simulink model "sm_water_powered_lift"  (R2026a)
settings: Solver=ode15s  StopTime=50  MaxStep=1e-2  AbsTol=1e-4  EnableMultiTasking=on
undefined symbols (not defined in the file or in its folder): wrat, X, Y, Z
libraries: sm_lib x47, nesl_utility x13, fl_lib x10, Multibody_Parts_Lib x2, simulink x1
(part 1 of 2)
CloseFcn:
  | try,close(h1_sm_water_powered_lift),end
  | clear h1_sm_water_powered_lift
  | 
  | clear simlog_sm_water_powered_lift
  | clear logsout_sm_water_powered_lift
Description:
  | Water Powered Lift
  | 
  | Copyright 2017-2026 The MathWorks, Inc.
settings Model: Tag=PublishSubsystem  Creator=smiller  LastModifiedBy=smiller
settings DataIOCC: MaxDataPoints=15000  SignalLoggingName=logsout_sm_water_powered_lift
settings DebuggingCC: PregeneratedLibrarySubsystemCodeDiagnostic=none
settings SimscapeCC: SimscapeNormalizeSystem=off  SimscapeNominalValues="[{\"value\":\"1\",\"unit\":\"A\"},{\"value\":\"1\",\"unit\":\"bar\"},{\"value\":\"1\",\"unit\":\"cm^2\"},{\"value\":\"1\",\"unit\":\"cm^3/s\"},{\"value\":\"1\",\"unit\":\"kJ/kg\"},{\"value\":\"1\",\"unit\":\"kW\"},{\"value\":\"1\",\"unit\":\"l\"},{\"value\":\"1\",\"unit\":\"N\"},{\"value\":\"1\",\"unit\":\"N*m\"},{\"value\":\"1\",\"unit\":\"V\"}]"  SimscapeLogSimulationStatistics=on  SimscapeLogName=simlog_sm_water_powered_lift  SimscapeLogDataHistory=15000.0
settings ConfigurationSet: Description=SimMechanics 2G
settings ExplorerConfigSet: InternalSimMechanicsExplorerSettings="<ExplorerConfiguration><canonicalview>default</canonicalview><AnimationSetting><BasePlaybackSpeed>1.0</BasePlaybackSpeed><PlaybackSpeedFactor>2.0</PlaybackSpeedFactor></AnimationSetting><TilePanel><TileInfo><Tiles Columns=\"2\" Count=\"4\" Rows=\"2\"><Column Left=\"2\" Weight=\"0.4992\"/><Column Left=\"314\" Weight=\"0.5008\"/><Column Left=\"627\"/><Row Top=\"2\" Weight=\"0.4993\"/><Row Top=\"345\" Weight=\"0.5007\"/><Row Top=\"689\"/><Tile Height=\"1\" Width=\"1\" X=\"0\" Y=\"0\"/><Tile Height=\"1\" Width=\"1\" X=\"0\" Y=\"1\"/><Tile Height=\"1\" Width=\"1\" X=\"1\" Y=\"0\"/><Tile Height=\"1\" Width=\"1\" X=\"1\" Y=\"1\"/></Tiles></TileInfo><SceneInfo><SceneViewer><BGColor><R>1</R><G>1</G><B>1</B></BGColor><Camera><DoPerspective>off</DoPerspective><Position><X>-0.33865632822427127</X><Y>-0.74181965766312075</Y><Z>0.63517646256957694</Z></Position><Center><X>0.17435806215764543</X><Y>0.41659149528563333</Y><Z>0.46311042540191633</Z></Center><Up><X>0.044233510300130147</X><Y>0.12758646822646313</Y><Z>0.99084059751910947</Z></Up><ViewLimDist>1</ViewLimDist><YLim>0.73418943875669118</YLim><XLim>0.66604610761460303</XLim></Camera></SceneViewer><SceneViewer><BGColor><R>1</R><G>1</G><B>1</B></BGColor><Camera><DoPerspective>on</DoPerspective><Position><X>-0.36750000000000016</X><Y>0.94385156136048332</Y><Z>0.52251828153286128</Z></Position><Center><X>-0.12000000000000008</X><Y>0.94875767701724301</Y><Z>0.32382884414586155</Z></Center><Up><X>0</X><Y>0</Y><Z>1</Z></Up><ViewLimDist>1</ViewLimDist><YLim>0.46630765815499858</YLim><XLim>0.42176483707750617</XLim></Camera></SceneViewer><SceneViewer><BGColor><R>1</R><G>1</G><B>1</B></BGColor><Camera><DoPerspective>off</DoPerspective><Position><X>-0.8984869340885806</X><Y>0.0036381965185360507</Y><Z>0.11209190037180658</Z></Position><Center><X>0.20238156217890113</X><Y>0.0036381965185360507</Y><Z>0.11209190037180658</Z></Center><Up><X>0</X><Y>0</Y><Z>1</Z></Up><ViewLimDist>1</ViewLimDist><YLim>0.37360343949453689</YLim><XLim>0.34004624433035691</XLim></Camera></SceneViewer><SceneViewer><BGColor><R>1</R><G>1</G><B>1</B></BGColor><Camera><DoPerspective>on</DoPerspective><Position><X>0.10106831738082762</X><Y>-0.30413148543864094</Y><Z>0.35203766090491534</Z></Position><Center><X>0.3950004490262965</X><Y>-0.032632326314832705</Y><Z>0.15132570006540724</Z></Center><Up><X>0.30158145199882502</X><Y>0.33375611692514179</Y><Z>0.89311560406552715</Z></Up><ViewLimDist>1</ViewLimDist><YLim>0.46630765815499858</YLim><XLim>0.42315680023617785</XLim></Camera></SceneViewer></SceneInfo></TilePanel><MechEditorPanel><Cameras><Camera><Id>Camera1</Id><Value><Name>Bucket</Name><NativeCamera><PositionTrackingFeature>Arm.Bucket.Transform_Camera.F</PositionTrackingFeature><CenterTrackingFeature>Arm.Arm.Pin_Side_1.Frame1</CenterTrackingFeature><UpVectorTrackingFeature>World_Frame.W</UpVectorTrackingFeature><CenterTrackingOrigin>on</CenterTrackingOrigin><UpVectorTrackingDirection>+Z</UpVectorTrackingDirection></NativeCamera></Value></Camera><Camera><Id>Camera2</Id><Value><Name>Gear</Name><NativeCamera><PositionKeyframeSet><Keyframe><Time>+0.0000000000000000e+00</Time><Value><X>+1.0106831738082762e-01</X><Y>-3.0413148543864094e-01</Y><Z>+3.5203766090491534e-01</Z></Value></Keyframe></PositionKeyframeSet><CenterKeyframeSet><Keyframe><Time>+0.0000000000000000e+00</Time><Value><X>+3.9500044902629650e-01</X><Y>-3.2632326314832705e-02</Y><Z>+1.5132570006540724e-01</Z></Value></Keyframe></CenterKeyframeSet><UpVectorKeyframeSet><Keyframe><Time>+0.0000000000000000e+00</Time><Value><X>+3.0158145199882502e-01</X><Y>+3.3375611692514179e-01</Y><Z>+8.9311560406552715e-01</Z></Value></Keyframe></UpVectorKeyframeSet></NativeCamera></Value></Camera></Cameras><GfxPanelCameraMap><MapElement CameraMLId=\"Camera1\" GfxPanelIndex=\"1\"/><MapElement CameraMLId=\"Camera2\" GfxPanelIndex=\"3\"/></GfxPanelCameraMap><VideoCreator><PlaybackSpeedRatio>1.0</PlaybackSpeedRatio><FrameRate>30</FrameRate><VideoFormat>Motion JPEG AVI</VideoFormat><FrameSize>auto</FrameSize></VideoCreator></MechEditorPanel></ExplorerConfiguration>"

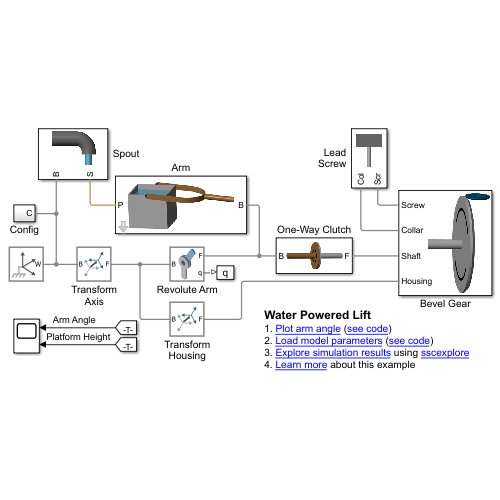
[thumbnail: Simulink's stored preview of the top-level diagram]
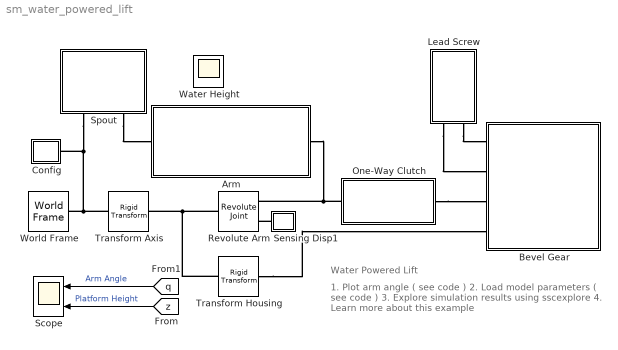
== system sm_water_powered_lift ==
  note: Water Powered Lift
  note: 1. Plot arm angle ( see code )
      | 2. Load model parameters ( see code )
      | 3. Explore simulation results using sscexplore
      | 4. Learn more about this example
  Arm : Subsystem  mask(Water Wheel Arm with Bucket){spoke_angle=30, spoke_length=wrat.spoke.length, spoke_radius=wrat.spoke.radius, spoke_angle_fill=-[40 55], bracket_rad=wrat.bracket.radius, bracket_height=wrat.bracket.height, bracket_thickness=wrat.bracket.thickness, bracket_sidelen=wrat.bracket.side.length, arc_xc=wrat.bracket.extr_data, whl_rho=wrat.wheel.rho, whl_clr=wrat.wheel.color, bucket_side=wrat.bucket.side, bucket_height=wrat.bucket.height, bucket_hole_side=wrat.bucket.hole.side, pin_viscfrict=wrat.bucket.pin_friction, bucket_rho=wrat.bucket.rho, bucket_wallthickness=wrat.bucket.wall_thickness, bucket_clr=wrat.bucket.color, bucket_opc=wrat.bucket.opacity*0.5, water_rho=wrat.water.rho, check_wlevel=off, water_clr_level=wrat.water.clr, water_opc_level=wrat.water.opc, water_thickness_level=wrat.water.surface_thickness, check_wellip=off, water_clr_ellip=wrat.water.clr, water_opc_ellip=wrat.water.opc}
      mask prompts: spoke_angle "Angle (deg)"; spoke_length "Length (m)"; spoke_radius "Radius (m)"; spoke_angle_fill "Angle Range for Fill [min max] (deg)"; bracket_rad "Radius (m)"; bracket_height "Height (m)"; bracket_thickness "Thickness (m)"; bracket_sidelen "Side Length (m)"; arc_xc "Arc Cross Section [xy] (m)"; whl_rho "Density (kg/m^3)"; whl_clr "Color [RGB]"; bucket_side "Side Length (m)"; bucket_height "Height (m)"; bucket_hole_side "Hole Side Length (m)"; pin_viscfrict "Friction at Pin (N*m/(deg/s))"; bucket_rho "Density (kg/m^3)"; bucket_wallthickness "Wall Thickness (m)"; bucket_clr "Color [RGB]"; bucket_opc "Opacity (0-1)"; water_rho "Density (kg/m^3)"; check_wlevel "Show Water Level"; water_clr_level "Color [RGB]"; water_opc_level "Opacity (0-1)"; water_thickness_level "Surface thickness (m)"; check_wellip "Show Water Inertia Ellipsoid"; water_clr_ellip "Color [RGB]"; water_opc_ellip "Opacity (0-1)"
      mask help: Models a single spoke of a water wheel with a bucket at the end. Multibody port B is the axis end of the arm. Inport Flow is the volumetric flow of water in kg^3/s.
      mask init:
      | bucket_wall_xc =[
      |     bucket_side/2  bucket_side/2;
      |     -bucket_side/2  bucket_side/2;
      |     -bucket_side/2  -bucket_side/2;
      |     bucket_side/2  -bucket_side/2;
      |     bucket_side/2  bucket_side/2;
      |     bucket_side/2-bucket_wallthickness  bucket_side/2-bucket_wallthickness;
      |     bucket_side/2-bucket_wallthickness  -(bucket_side/2-bucket_wallthickness);
      |     -(bucket_side/2-bucket_wallthickness)  -(bucket_side/2-bucket_wallthickness);
      |     -(bucket_side/2-bucket_wallthickness)  (bucket_side/2-bucket_wallthickness);
      |     (bucket_side/2-bucket_wallthickness)  (bucket_side/2-bucket_wallthickness)];
      | 
      | bucket_floor_xc = [
      |     bucket_side/2  bucket_side/2;
      |     -bucket_side/2  bucket_side/2;
      |     -bucket_side/2  -bucket_side/2;
      |     bucket_side/2  -bucket_side/2;
      |     bucket_side/2  bucket_side/2;
      |     bucket_hole_side/2  bucket_hole_side/2;
      |     bucket_hole_side/2  -bucket_hole_side/2;
      |     -bucket_hole_side/2  -bucket_hole_side/2;
      |     -bucket_hole_side/2  bucket_hole_side/2;
      |     bucket_hole_side/2  bucket_hole_side/2];
      | 
      | f    = Simulink.FindOptions('FollowLinks',1,'LookUnderMasks','all');
      | wsv_h = Simulink.findBlocks(bdroot,'Name','Water Surface',f);
      | 
      | %wsv_h = char(find_system(gcb,'FollowLinks','on','LookUnderMasks','all','Name','Water Surface'));
      | if(check_wlevel)
      |     set_param(wsv_h,'OverrideUsingVariant','Show');
      | else
      | 	set_param(wsv_h,'OverrideUsingVariant','None');
      | end
      mask Callback check_wlevel:
      | maskObj = Simulink.Mask.get(gcb);
      | cont_waterlevel_h = maskObj.getDialogControl('cont_waterlevel');
      | 
      | temp_showwaterlevel = get_param(gcb,'check_wlevel');
      | cont_waterlevel_h.Visible = temp_showwaterlevel;
      | 
      | clear maskObj temp_showwaterlevel cont_waterlevel_h
      mask Callback check_wellip:
      | maskObj = Simulink.Mask.get(gcb);
      | cont_waterellipsoid_h = maskObj.getDialogControl('cont_waterellipsoid');
      | 
      | temp_showwaterellipsoid = get_param(gcb,'check_wellip');
      | cont_waterellipsoid_h.Visible = temp_showwaterellipsoid;
      | 
      | clear maskObj temp_showwaterellipsoid cont_waterellipsoid_h
      mask DialogControl cont_spoke Prompt: Spoke
      mask DialogControl cont_bracket Prompt: Bracket
      mask DialogControl cont_wheel Prompt: Wheel
      mask DialogControl cont_bucket Prompt: Bucket
      mask DialogControl cont_water Prompt: Water
      mask DialogControl cont_waterlevel Prompt: Water Level Visual
      mask DialogControl cont_waterellipsoid Prompt: Water Inertia Ellipsoid
      mask Display: image('sm_water_powered_lift_arm_IMAGE.png');
  Bevel Gear : Subsystem
      mask Display: image('sm_water_powered_lift_bevel_gear_IMAGE.png');
  Config : Subsystem
  Lead Screw : Subsystem
      mask Display: image('sm_water_powered_lift_lead_screw_IMAGE.png');
  One-Way Clutch : Subsystem
      mask Display: image('sm_water_powered_lift_one_way_clutch_IMAGE.png');
  Revolute Arm : sm_lib/Joints/Revolute Joint  JointMode=Normal  CompositeWrenchDir=FollowerOnBase  CompositeWrenchFrame=BaseFrame  SenseConstraintForce=off  SenseConstraintTorque=off  SenseTotalForce=off  SenseTotalTorque=off  PositionTargetSpecify=on  PositionTargetPriority=High  PositionTargetValue=0  PositionTargetValueUnits=deg  VelocityTargetSpecify=off  VelocityTargetPriority=High  VelocityTargetValue=0  VelocityTargetValueUnits=deg/s  EquilibriumPosition=wrat.spring.equilib_pos-30  EquilibriumPositionUnits=deg  SpringStiffness=wrat.spring.stiffness  SpringStiffnessUnits=N*m/deg  DampingCoefficient=wrat.spring.damping  DampingCoefficientUnits=N*m/(deg/s)  LowerLimitSpecify=off  LowerLimitBound=-90  LowerLimitBoundUnits=deg  LowerLimitStiffness=1e4  LowerLimitStiffnessUnits=N*m/deg  LowerLimitDamping=10  LowerLimitDampingUnits=N*m/(deg/s)  LowerLimitTransitionRegionWidth=0.1  LowerLimitTransitionRegionWidthUnits=deg  UpperLimitSpecify=off  UpperLimitBound=90  UpperLimitBoundUnits=deg  UpperLimitStiffness=1e4  UpperLimitStiffnessUnits=N*m/deg  UpperLimitDamping=10  UpperLimitDampingUnits=N*m/(deg/s)  UpperLimitTransitionRegionWidth=0.1  UpperLimitTransitionRegionWidthUnits=deg  TorqueActuationMode=NoTorque  MotionActuationMode=ComputedMotion  SensePosition=on  SenseVelocity=off  SenseAcceleration=off  SenseTorqueForce=off  SenseLowerLimitTorqueForce=off  SenseUpperLimitTorqueForce=off
  Scope : Scope  NumInputPorts=2
      settings: ActiveDisplayYMinimum=-18.72034  ActiveDisplayYMaximum=24.90299
  Sensing Disp1 : Subsystem
      mask Display: disp('q')
  Spout : Subsystem
      mask Display: image('sm_water_powered_lift_spout_IMAGE.png');
  Transform Axis : sm_lib/Frames and Transforms/Rigid Transform  RotationMethod=StandardAxis  FollAlignAxisA=+X  BaseAlignAxisA=+Y  FollAlignAxisB=+Y  BaseAlignAxisB=+Z  RotationStandardAxis=+Y  RotationAngle=90  RotationAngleUnits=deg  RotationArbitraryAxis=[0 0 1]  RotationSequenceAxes=FollowerAxes  RotationSequence=XYX  RotationSequenceAngles=[0 0 0]  RotationSequenceAnglesUnits=deg  RotationMatrix=[1 0 0; 0 1 0; 0 0 1]  Quaternion=[1 0 0 0]  TranslationMethod=None  TranslationCartesianOffset=[0 0 0]  TranslationCartesianOffsetUnits=m  TranslationStandardAxis=+Z  TranslationStandardOffset=0  TranslationStandardOffsetUnits=m  TranslationROffset=0  TranslationROffsetUnits=m  TranslationThetaOffset=0  TranslationThetaOffsetUnits=deg  TranslationZOffset=0  TranslationZOffsetUnits=m
  Transform Housing : sm_lib/Frames and Transforms/Rigid Transform  RotationMethod=StandardAxis  FollAlignAxisA=+X  BaseAlignAxisA=+Y  FollAlignAxisB=+Y  BaseAlignAxisB=+Z  RotationStandardAxis=+Z  RotationAngle=180  RotationAngleUnits=deg  RotationArbitraryAxis=[0 0 1]  RotationSequenceAxes=FollowerAxes  RotationSequence=XYX  RotationSequenceAngles=[0 0 0]  RotationSequenceAnglesUnits=deg  RotationMatrix=[1 0 0; 0 1 0; 0 0 1]  Quaternion=[1 0 0 0]  TranslationMethod=StandardAxis  TranslationCartesianOffset=[0 0 0]  TranslationCartesianOffsetUnits=m  TranslationStandardAxis=+Z  TranslationStandardOffset=0.4  TranslationStandardOffsetUnits=m  TranslationROffset=0  TranslationROffsetUnits=m  TranslationThetaOffset=0  TranslationThetaOffsetUnits=deg  TranslationZOffset=0  TranslationZOffsetUnits=m
  World Frame : sm_lib/Frames and Transforms/World Frame
  Water Height : Scope
      settings: ActiveDisplayYMinimum=-0.02344  ActiveDisplayYMaximum=0.21094
  wires:
  [z] -> Scope/2  "Platform Height"
  [q] -> Scope/1  "Arm Angle"
  connections:
  Revolute Arm/LConn1 -- Transform Housing/LConn1 -- Transform Axis/RConn1
  Transform Housing/RConn1 -- Bevel Gear/LConn4
  Sensing Disp1/LConn1 -- Revolute Arm/RConn2
  World Frame/RConn1 -- Config/LConn1 -- Spout/LConn1 -- Transform Axis/LConn1
  Lead Screw/RConn2 -- Bevel Gear/LConn1
  Lead Screw/RConn1 -- Bevel Gear/LConn2
  Spout/LConn2 -- Arm/LConn1
  Arm/RConn1 -- One-Way Clutch/LConn1 -- Revolute Arm/RConn1
  One-Way Clutch/RConn1 -- Bevel Gear/LConn3

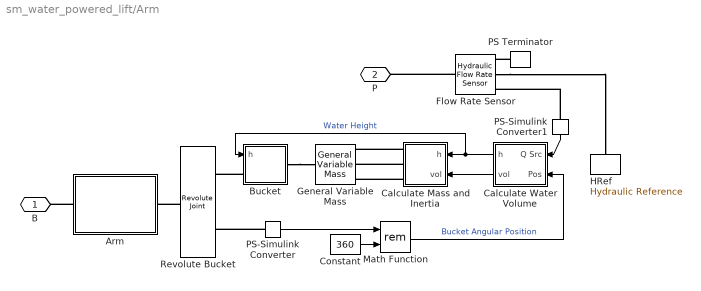
== system sm_water_powered_lift/Arm ==
  Arm : Subsystem
  Bucket : Subsystem
  Calculate Mass and Inertia : Subsystem
  Calculate Water Volume : Subsystem
  Constant : Constant  Value=360
  Flow Rate Sensor : fl_lib/Hydraulic/Hydraulic Sensors/Hydraulic Flow Rate Sensor
  General Variable Mass : sm_lib/Body Elements/Variable Mass/General Variable Mass  VariableInertiaType=Custom  MassType=TimeVarying  Mass=1  MassUnits=kg  CenterOfMassType=TimeVarying  CenterOfMass=[0 0 0]  CenterOfMassUnits=m  InertiaMatrixType=TimeVarying  MomentsOfInertia=[1 1 1]*0.01  MomentsOfInertiaUnits=kg*m^2  ProductsOfInertia=[0 0 0]  ProductsOfInertiaUnits=kg*m^2  GraphicType=InertiaEllipsoid  MarkerShape=Sphere  MarkerSize=10  GraphicVisPropType=SimpleVisualProperties  GraphicDiffuseColor=water_clr_ellip  GraphicOpacity=water_opc_ellip*check_wellip  GraphicSpecularColor=[0.5 0.5 0.5 1.0]  GraphicAmbientColor=[0.15 0.15 0.15 1.0]  GraphicEmissiveColor=[0.0 0.0 0.0 1.0]  GraphicShininess=75
  HRef : fl_lib/Hydraulic/Hydraulic Elements/Hydraulic Reference
  Math Function : Math  Operator=rem  SignedPower=on
  PS Terminator : fl_lib/Physical Signals/Sinks/PS Terminator
  PS-Simulink Converter : nesl_utility/PS-Simulink Converter  PhysicalDomain=network_engine_domain  SubClassName=ps_output  LeftPortType=input  RightPortType=output  PseudoPeriodic=off  Frequencies=[]  VectorFormat=1-D array  Unit=deg  AffineConversion=off
  PS-Simulink Converter1 : nesl_utility/PS-Simulink Converter  PhysicalDomain=network_engine_domain  SubClassName=ps_output  LeftPortType=input  RightPortType=output  PseudoPeriodic=off  Frequencies=[]  VectorFormat=1-D array  Unit=m^3/s  AffineConversion=off
  Revolute Bucket : sm_lib/Joints/Revolute Joint  JointMode=Normal  CompositeWrenchDir=FollowerOnBase  CompositeWrenchFrame=BaseFrame  SenseConstraintForce=off  SenseConstraintTorque=off  SenseTotalForce=off  SenseTotalTorque=off  PositionTargetSpecify=on  PositionTargetPriority=High  PositionTargetValue=-spoke_angle  PositionTargetValueUnits=deg  VelocityTargetSpecify=off  VelocityTargetPriority=High  VelocityTargetValue=0  VelocityTargetValueUnits=deg/s  EquilibriumPosition=0  EquilibriumPositionUnits=deg  SpringStiffness=0  SpringStiffnessUnits=N*m/deg  DampingCoefficient=pin_viscfrict  DampingCoefficientUnits=N*m/(deg/s)  LowerLimitSpecify=off  LowerLimitBound=-90  LowerLimitBoundUnits=deg  LowerLimitStiffness=1e4  LowerLimitStiffnessUnits=N*m/deg  LowerLimitDamping=10  LowerLimitDampingUnits=N*m/(deg/s)  LowerLimitTransitionRegionWidth=0.1  LowerLimitTransitionRegionWidthUnits=deg  UpperLimitSpecify=off  UpperLimitBound=90  UpperLimitBoundUnits=deg  UpperLimitStiffness=1e4  UpperLimitStiffnessUnits=N*m/deg  UpperLimitDamping=10  UpperLimitDampingUnits=N*m/(deg/s)  UpperLimitTransitionRegionWidth=0.1  UpperLimitTransitionRegionWidthUnits=deg  TorqueActuationMode=NoTorque  MotionActuationMode=ComputedMotion  SensePosition=on  SenseVelocity=off  SenseAcceleration=off  SenseTorqueForce=off  SenseLowerLimitTorqueForce=off  SenseUpperLimitTorqueForce=off
  B : PMIOPort  Side=Right
  P : PMIOPort  Port=2  Side=Left
  wires:
  PS-Simulink Converter/1 -> Math Function/1
  Calculate Water Volume/1(h) -> Calculate Mass and Inertia/1(h), Bucket/1(h)  "Water Height"
  Constant/1 -> Math Function/2
  Math Function/1 -> Calculate Water Volume/2(Pos)  "Bucket Angular Position"
  Calculate Water Volume/2(vol) -> Calculate Mass and Inertia/2(vol)
  PS-Simulink Converter1/1 -> Calculate Water Volume/1(Q Src)
  connections:
  PS-Simulink Converter/LConn1 -- Revolute Bucket/RConn2
  Bucket/RConn1 -- General Variable Mass/RConn1
  Bucket/LConn1 -- Revolute Bucket/RConn1
  Arm/LConn1 -- B/RConn1
  Revolute Bucket/LConn1 -- Arm/RConn1
  Calculate Mass and Inertia/RConn1 -- General Variable Mass/LConn1
  Calculate Mass and Inertia/RConn2 -- General Variable Mass/LConn2
  Calculate Mass and Inertia/RConn3 -- General Variable Mass/LConn3
  Flow Rate Sensor/LConn1 -- P/RConn1
  PS-Simulink Converter1/LConn1 -- Flow Rate Sensor/RConn1
  PS Terminator/LConn1 -- Flow Rate Sensor/RConn3
  Flow Rate Sensor/RConn2 -- HRef/LConn1

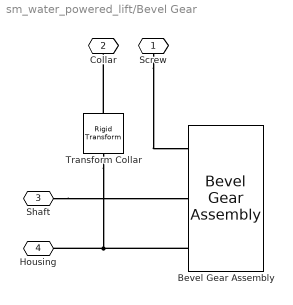
== system sm_water_powered_lift/Bevel Gear ==
  Bevel Gear Assembly : Multibody_Parts_Lib/Gears/Assemblies/Bevel Gear Assembly  Tag=PublishSubsystem  bevel_angle_asy=90  b_cone_angle_asy=90/2  b_radius_asy=wrat.gear.drive.radius  f_radius_asy=wrat.gear.out.radius  b_thickness_asy=wrat.gear.drive.len*2  f_thickness_asy=wrat.gear.out.len  b_hole_radius_asy=wrat.gear_shaft.rad  f_hole_radius_asy=wrat.screw.radius  b_rho_asy=7000  f_rho_asy=7000  b_clr_asy=wrat.gear.drive.clr  f_clr_asy=wrat.gear.out.clr  b_opc_asy=1  f_opc_asy=1  b_visc_frict_asy=0.1  f_visc_frict_asy=0.1  b_popup_markings=Two  f_popup_markings=Two  b_mark_radius_range=[0.7 0.75]  f_mark_radius_range=[0.6 0.75]  b_mark_angle_range=120  f_mark_angle_range=120  b_mark_clr=[0 0 0]  f_mark_clr=[1 1 1]
      settings: SourceProductName=Simscape Multibody Parts Library
  Transform Collar : sm_lib/Frames and Transforms/Rigid Transform  RotationMethod=StandardAxis  FollAlignAxisA=+X  BaseAlignAxisA=+Y  FollAlignAxisB=+Y  BaseAlignAxisB=+Z  RotationStandardAxis=+Y  RotationAngle=-90  RotationAngleUnits=deg  RotationArbitraryAxis=[0 0 1]  RotationSequenceAxes=FollowerAxes  RotationSequence=XYX  RotationSequenceAngles=[0 0 0]  RotationSequenceAnglesUnits=deg  RotationMatrix=[1 0 0; 0 1 0; 0 0 1]  Quaternion=[1 0 0 0]  TranslationMethod=Cartesian  TranslationCartesianOffset=[wrat.gear.drive.radius 0 wrat.gear.out.radius]  TranslationCartesianOffsetUnits=m  TranslationStandardAxis=+Z  TranslationStandardOffset=0  TranslationStandardOffsetUnits=m  TranslationROffset=0  TranslationROffsetUnits=m  TranslationThetaOffset=0  TranslationThetaOffsetUnits=deg  TranslationZOffset=0  TranslationZOffsetUnits=m
  Screw : PMIOPort  Side=Left
  Collar : PMIOPort  Port=2  Side=Left
  Shaft : PMIOPort  Port=3  Side=Left
  Housing : PMIOPort  Port=4  Side=Left
  connections:
  Bevel Gear Assembly/LConn3 -- Housing/RConn1 -- Transform Collar/LConn1
  Shaft/RConn1 -- Bevel Gear Assembly/LConn2
  Screw/RConn1 -- Bevel Gear Assembly/LConn1
  Transform Collar/RConn1 -- Collar/RConn1

== system sm_water_powered_lift/Config ==
  Mechanism Configuration : sm_lib/Utilities/Mechanism Configuration  UniformGravity=Constant  GravityVector=[0 0 -9.80665]  GravityVectorUnits=m/s^2  LinearizationDelta=0.001  JointModeTransitionNonlinearIterations=2
  Solver Configuration : nesl_utility/Solver Configuration  PhysicalDomain=network_engine_domain  SubClassName=solver  LeftPortType=input  RightPortType=generic  Tones=[]  Harmonics=[]  SimulateNoise=off  Profile=off  UseLocalSampling=off  EnableSwitchedLinearOptims=on  FrequencyDomain=off  UseCCode=off  RelTol=0.001  AbsTol=1e-06  MinStep=1e-09  ToWorkspace=off  RevertToSquareIcSolve=off  NumHomotopyIterations=100  PhasorMode=off  PhasorModeNumHarmonics=1  ConsistencySolver=NEWTON_FTOL  CanonicalOrdering=UNORDERED  OptimizeIntermediates=UNOPTIMIZED  IndexReductionMethod=DerivativeReplacement  DoDC=off  ResidualTolerance=1e-09  ConsistencyTolSource=GLOBAL  ConsistencyAbsTol=0.001  ConsistencyRelTol=0.001  ConsistencyTolFactor=0.001  UseLocalSolver=off  LocalSolverChoice=NE_BACKWARD_EULER_ADVANCER  ResolveIndetEquations=on  FunctionEvalNumThread=1  LocalSolverSampleTime=0.001  DoFixedCost=off  MaxNonlinIter=3  MaxModeIter=2  ComputeImpulses=off  ImpulseIterations=2  LinearAlgebra=Sparse  LinearAlgebraNumThread=0  EquationFormulation=NE_TIME_EF  DelaysMemoryBudget=1024  AutomaticFiltering=on  FilteringTimeConstant=0.001  PartitionStorageMethod=AS_NEEDED  PartitionMemoryBudget=1024  PartitionMethod=FAST  MultibodyUseLocalSolver=off  MultibodyLocalSolverChoice=ODE1  MultibodyLocalSolverSampleTime=0.001
  C : PMIOPort  Side=Left
  connections:
  Mechanism Configuration/RConn1 -- C/RConn1 -- Solver Configuration/RConn1

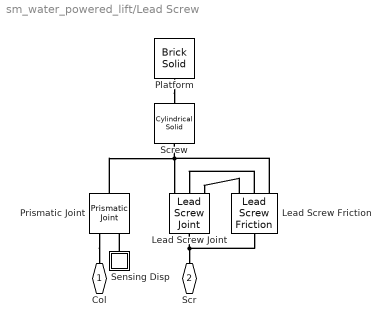
== system sm_water_powered_lift/Lead Screw ==
  Lead Screw Joint : sm_lib/Joints/Lead Screw Joint  JointMode=Normal  CompositeWrenchDir=FollowerOnBase  CompositeWrenchFrame=BaseFrame  SenseConstraintForce=on  SenseConstraintTorque=off  SenseTotalForce=off  SenseTotalTorque=off  Direction=RightHand  Lead=wrat.screw.lead  LeadUnits=m/rev  PositionTargetSpecify=off  PositionTargetPriority=High  PositionTargetRotationBased=off  PositionTargetRotationValue=0  PositionTargetRotationValueUnits=deg  PositionTargetTranslationValue=0  PositionTargetTranslationValueUnits=m  VelocityTargetSpecify=off  VelocityTargetPriority=High  VelocityTargetRotationBased=off  VelocityTargetRotationValue=0  VelocityTargetRotationValueUnits=deg/s  VelocityTargetTranslationValue=0  VelocityTargetTranslationValueUnits=m/s  SenseRotationPosition=off  SenseRotationVelocity=on  SenseRotationAcceleration=off  SenseTranslationPosition=off  SenseTranslationVelocity=off  SenseTranslationAcceleration=off
  Lead Screw Friction : Multibody_Parts_Lib/Gears/Forces/Lead Screw Friction  Tag=PublishSubsystem  mu_kinetic=wrat.screw.muk  mu_static=wrat.screw.mus  vel_th=1e-3  lead=wrat.screw.lead  screw_radius=wrat.screw.radius  filt_const=1e-3
      settings: SourceProductName=Simscape Multibody Parts Library
      settings: AttributesFormatString=|
      | Lead Angle =  deg
      | Kinetic Friction =
  Platform : sm_lib/Body Elements/Brick Solid  BrickDimensions=[0.2 0.2 0.1]  BrickDimensionsUnits=m  ExportEntireGeometry=off  InertiaType=CalculateFromGeometry  BasedOnType=Density  Density=1000  DensityUnits=kg/m^3  Mass=1  MassUnits=kg  CenterOfMass=[0 0 0]  CenterOfMassUnits=m  MomentsOfInertia=[1 1 1]  MomentsOfInertiaUnits=kg*m^2  ProductsOfInertia=[1 1 1]  ProductsOfInertiaUnits=kg*m^2  GraphicType=FromGeometry  MarkerShape=Sphere  MarkerSize=10  GraphicVisPropType=SimpleVisualProperties  GraphicDiffuseColor=[0.5 0.5 0.5]  GraphicOpacity=1.0  GraphicSpecularColor=[0.5 0.5 0.5 1.0]  GraphicAmbientColor=[0.15 0.15 0.15 1.0]  GraphicEmissiveColor=[0.0 0.0 0.0 1.0]  GraphicShininess=75  DoExposeReferenceFrame=on  SerializedFrames=<Frames/>
  Prismatic Joint : sm_lib/Joints/Prismatic Joint  JointMode=Normal  CompositeWrenchDir=FollowerOnBase  CompositeWrenchFrame=BaseFrame  SenseConstraintForce=off  SenseConstraintTorque=off  SenseTotalForce=off  SenseTotalTorque=off  PositionTargetSpecify=off  PositionTargetPriority=High  PositionTargetValue=0  PositionTargetValueUnits=m  VelocityTargetSpecify=off  VelocityTargetPriority=High  VelocityTargetValue=0  VelocityTargetValueUnits=m/s  EquilibriumPosition=0  EquilibriumPositionUnits=m  SpringStiffness=0  SpringStiffnessUnits=N/m  DampingCoefficient=0  DampingCoefficientUnits=N/(m/s)  LowerLimitSpecify=off  LowerLimitBound=-1  LowerLimitBoundUnits=m  LowerLimitStiffness=1e6  LowerLimitStiffnessUnits=N/m  LowerLimitDamping=1e3  LowerLimitDampingUnits=N/(m/s)  LowerLimitTransitionRegionWidth=1e-4  LowerLimitTransitionRegionWidthUnits=m  UpperLimitSpecify=off  UpperLimitBound=1  UpperLimitBoundUnits=m  UpperLimitStiffness=1e6  UpperLimitStiffnessUnits=N/m  UpperLimitDamping=1e3  UpperLimitDampingUnits=N/(m/s)  UpperLimitTransitionRegionWidth=1e-4  UpperLimitTransitionRegionWidthUnits=m  TorqueActuationMode=NoTorque  MotionActuationMode=ComputedMotion  SensePosition=on  SenseVelocity=off  SenseAcceleration=off  SenseTorqueForce=off  SenseLowerLimitTorqueForce=off  SenseUpperLimitTorqueForce=off
  Screw : sm_lib/Body Elements/Cylindrical Solid  CylinderRadius=wrat.screw.radius  CylinderRadiusUnits=m  CylinderLength=wrat.screw.length  CylinderLengthUnits=m  ExportEntireGeometry=off  InertiaType=CalculateFromGeometry  BasedOnType=Density  Density=1000  DensityUnits=kg/m^3  Mass=1  MassUnits=kg  CenterOfMass=[0 0 0]  CenterOfMassUnits=m  MomentsOfInertia=[1 1 1]  MomentsOfInertiaUnits=kg*m^2  ProductsOfInertia=[1 1 1]  ProductsOfInertiaUnits=kg*m^2  GraphicType=FromGeometry  MarkerShape=Sphere  MarkerSize=10  GraphicVisPropType=SimpleVisualProperties  GraphicDiffuseColor=[0.8 0.8 0.8]  GraphicOpacity=1.0  GraphicSpecularColor=[0.5 0.5 0.5 1.0]  GraphicAmbientColor=[0.15 0.15 0.15 1.0]  GraphicEmissiveColor=[0.0 0.0 0.0 1.0]  GraphicShininess=75  DoExposeReferenceFrame=on  SerializedFrames=<Frames><Frame><Id>Frame1</Id><Value><Name>T</Name><Origin><Source>GeometricFeature</Source><FeatureName>bottom surface</FeatureName></Origin><PrimaryAxis><DefinedDirection>+Z</DefinedDirection><Source>ReferenceFrame</Source><SourceDirection>+Z</SourceDirection><FeatureName></FeatureName></PrimaryAxis><SecondaryAxis><DefinedDirection>+X</DefinedDirection><Source>ReferenceFrame</Source><SourceDirection>+X</SourceDirection><FeatureName></FeatureName></SecondaryAxis></Value></Frame></Frames>
  Sensing Disp : Subsystem
      mask Display: disp('z')
  Col : PMIOPort  Side=Right
  Scr : PMIOPort  Port=2  Side=Right
  connections:
  Prismatic Joint/LConn1 -- Lead Screw Friction/LConn3 -- Screw/RConn1 -- Lead Screw Joint/RConn1
  Platform/RConn1 -- Screw/LConn1
  Lead Screw Friction/LConn1 -- Lead Screw Joint/RConn3
  Lead Screw Friction/LConn2 -- Lead Screw Joint/RConn2
  Lead Screw Joint/LConn1 -- Lead Screw Friction/RConn1 -- Scr/RConn1
  Prismatic Joint/RConn1 -- Col/RConn1
  Sensing Disp/LConn1 -- Prismatic Joint/RConn2

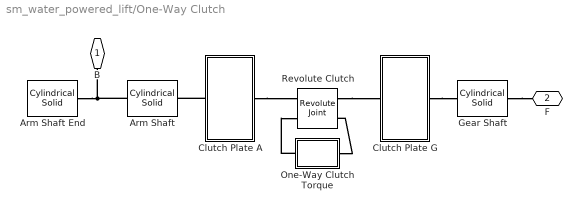
== system sm_water_powered_lift/One-Way Clutch ==
  Arm Shaft : sm_lib/Body Elements/Cylindrical Solid  CylinderRadius=wrat.arm_shaft.rad  CylinderRadiusUnits=m  CylinderLength=wrat.arm_shaft.len  CylinderLengthUnits=m  ExportEntireGeometry=off  InertiaType=CalculateFromGeometry  BasedOnType=Density  Density=1000  DensityUnits=kg/(m^3)  Mass=1  MassUnits=kg  CenterOfMass=[0 0 0]  CenterOfMassUnits=m  MomentsOfInertia=[1 1 1]  MomentsOfInertiaUnits=kg*m^2  ProductsOfInertia=[0 0 0]  ProductsOfInertiaUnits=kg*m^2  GraphicType=FromGeometry  MarkerShape=Sphere  MarkerSize=10  GraphicVisPropType=SimpleVisualProperties  GraphicDiffuseColor=wrat.wheel.color  GraphicOpacity=1.0  GraphicSpecularColor=[0.5 0.5 0.5 1.0]  GraphicAmbientColor=[0.15 0.15 0.15 1.0]  GraphicEmissiveColor=[0.0 0.0 0.0 1.0]  GraphicShininess=75  DoExposeReferenceFrame=off  SerializedFrames=<Frames><Frame><Id>Frame1</Id><Value><Name>Rtc</Name><Origin><Source>GeometricFeature</Source><FeatureName>top surface</FeatureName></Origin><PrimaryAxis><DefinedDirection>+Z</DefinedDirection><Source>ReferenceFrame</Source><SourceDirection>+Z</SourceDirection><FeatureName></FeatureName></PrimaryAxis><SecondaryAxis><DefinedDirection>+X</DefinedDirection><Source>ReferenceFrame</Source><SourceDirection>+X</SourceDirection><FeatureName></FeatureName></SecondaryAxis></Value></Frame><Frame><Id>Frame2</Id><Value><Name>Arm</Name><Origin><Source>GeometricFeature</Source><FeatureName>bottom surface</FeatureName></Origin><PrimaryAxis><DefinedDirection>+Z</DefinedDirection><Source>ReferenceFrame</Source><SourceDirection>+Z</SourceDirection><FeatureName></FeatureName></PrimaryAxis><SecondaryAxis><DefinedDirection>+X</DefinedDirection><Source>ReferenceFrame</Source><SourceDirection>+X</SourceDirection><FeatureName></FeatureName></SecondaryAxis></Value></Frame></Frames>
  Arm Shaft End : sm_lib/Body Elements/Cylindrical Solid  CylinderRadius=0.02  CylinderRadiusUnits=m  CylinderLength=0.02  CylinderLengthUnits=m  ExportEntireGeometry=off  InertiaType=CalculateFromGeometry  BasedOnType=Density  Density=1000  DensityUnits=kg/(m^3)  Mass=1  MassUnits=kg  CenterOfMass=[0 0 0]  CenterOfMassUnits=m  MomentsOfInertia=[1 1 1]  MomentsOfInertiaUnits=kg*m^2  ProductsOfInertia=[0 0 0]  ProductsOfInertiaUnits=kg*m^2  GraphicType=FromGeometry  MarkerShape=Sphere  MarkerSize=10  GraphicVisPropType=SimpleVisualProperties  GraphicDiffuseColor=wrat.wheel.color  GraphicOpacity=1.0  GraphicSpecularColor=[0.5 0.5 0.5 1.0]  GraphicAmbientColor=[0.15 0.15 0.15 1.0]  GraphicEmissiveColor=[0.0 0.0 0.0 1.0]  GraphicShininess=75  DoExposeReferenceFrame=off  SerializedFrames=<Frames><Frame><Id>Frame1</Id><Value><Name>Rtc</Name><Origin><Source>GeometricFeature</Source><FeatureName>top surface</FeatureName></Origin><PrimaryAxis><DefinedDirection>+Z</DefinedDirection><Source>ReferenceFrame</Source><SourceDirection>+Z</SourceDirection><FeatureName></FeatureName></PrimaryAxis><SecondaryAxis><DefinedDirection>+X</DefinedDirection><Source>ReferenceFrame</Source><SourceDirection>+X</SourceDirection><FeatureName></FeatureName></SecondaryAxis></Value></Frame></Frames>
  Clutch Plate A : Subsystem
      mask Display: image('sm_water_powered_lift_clutch_plate_a_IMAGE.png');
  Clutch Plate G : Subsystem
      mask Display: image('sm_water_powered_lift_clutch_plate_g_IMAGE.png');
  Gear Shaft : sm_lib/Body Elements/Cylindrical Solid  CylinderRadius=wrat.gear_shaft.rad  CylinderRadiusUnits=m  CylinderLength=wrat.gear_shaft.len  CylinderLengthUnits=m  ExportEntireGeometry=off  InertiaType=CalculateFromGeometry  BasedOnType=Density  Density=1000  DensityUnits=kg/(m^3)  Mass=1  MassUnits=kg  CenterOfMass=[0 0 0]  CenterOfMassUnits=m  MomentsOfInertia=[1 1 1]  MomentsOfInertiaUnits=kg*m^2  ProductsOfInertia=[0 0 0]  ProductsOfInertiaUnits=kg*m^2  GraphicType=FromGeometry  MarkerShape=Sphere  MarkerSize=10  GraphicVisPropType=SimpleVisualProperties  GraphicDiffuseColor=wrat.gear.drive.clr  GraphicOpacity=1.0  GraphicSpecularColor=[0.5 0.5 0.5 1.0]  GraphicAmbientColor=[0.15 0.15 0.15 1.0]  GraphicEmissiveColor=[0.0 0.0 0.0 1.0]  GraphicShininess=75  DoExposeReferenceFrame=off  SerializedFrames=<Frames><Frame><Id>Frame1</Id><Value><Name>Ge</Name><Origin><Source>GeometricFeature</Source><FeatureName>top surface</FeatureName></Origin><PrimaryAxis><DefinedDirection>+Z</DefinedDirection><Source>ReferenceFrame</Source><SourceDirection>+Z</SourceDirection><FeatureName></FeatureName></PrimaryAxis><SecondaryAxis><DefinedDirection>+X</DefinedDirection><Source>ReferenceFrame</Source><SourceDirection>+X</SourceDirection><FeatureName></FeatureName></SecondaryAxis></Value></Frame><Frame><Id>Frame2</Id><Value><Name>Rtc</Name><Origin><Source>GeometricFeature</Source><FeatureName>bottom surface</FeatureName></Origin><PrimaryAxis><DefinedDirection>+Z</DefinedDirection><Source>ReferenceFrame</Source><SourceDirection>+Z</SourceDirection><FeatureName></FeatureName></PrimaryAxis><SecondaryAxis><DefinedDirection>+X</DefinedDirection><Source>ReferenceFrame</Source><SourceDirection>+X</SourceDirection><FeatureName></FeatureName></SecondaryAxis></Value></Frame></Frames>
  One-Way Clutch Torque : Subsystem
  Revolute Clutch : sm_lib/Joints/Revolute Joint  JointMode=Normal  CompositeWrenchDir=FollowerOnBase  CompositeWrenchFrame=BaseFrame  SenseConstraintForce=off  SenseConstraintTorque=off  SenseTotalForce=off  SenseTotalTorque=off  PositionTargetSpecify=off  PositionTargetPriority=High  PositionTargetValue=0  PositionTargetValueUnits=deg  VelocityTargetSpecify=off  VelocityTargetPriority=High  VelocityTargetValue=0  VelocityTargetValueUnits=deg/s  EquilibriumPosition=0  EquilibriumPositionUnits=deg  SpringStiffness=0  SpringStiffnessUnits=N*m/deg  DampingCoefficient=0  DampingCoefficientUnits=N*m/(deg/s)  LowerLimitSpecify=off  LowerLimitBound=-90  LowerLimitBoundUnits=deg  LowerLimitStiffness=1e4  LowerLimitStiffnessUnits=N*m/deg  LowerLimitDamping=10  LowerLimitDampingUnits=N*m/(deg/s)  LowerLimitTransitionRegionWidth=0.1  LowerLimitTransitionRegionWidthUnits=deg  UpperLimitSpecify=off  UpperLimitBound=90  UpperLimitBoundUnits=deg  UpperLimitStiffness=1e4  UpperLimitStiffnessUnits=N*m/deg  UpperLimitDamping=10  UpperLimitDampingUnits=N*m/(deg/s)  UpperLimitTransitionRegionWidth=0.1  UpperLimitTransitionRegionWidthUnits=deg  TorqueActuationMode=InputTorque  MotionActuationMode=ComputedMotion  SensePosition=off  SenseVelocity=on  SenseAcceleration=off  SenseTorqueForce=off  SenseLowerLimitTorqueForce=off  SenseUpperLimitTorqueForce=off
  B : PMIOPort  Side=Left
  F : PMIOPort  Port=2  Side=Right
  connections:
  Gear Shaft/LConn1 -- F/RConn1
  Arm Shaft/RConn1 -- Arm Shaft End/LConn1 -- B/RConn1
  One-Way Clutch Torque/RConn1 -- Revolute Clutch/LConn2
  One-Way Clutch Torque/LConn1 -- Revolute Clutch/RConn2
  Clutch Plate A/LConn1 -- Arm Shaft/LConn1
  Clutch Plate A/RConn1 -- Revolute Clutch/LConn1
  Revolute Clutch/RConn1 -- Clutch Plate G/LConn1
  Clutch Plate G/RConn1 -- Gear Shaft/RConn1

== system sm_water_powered_lift/Sensing Disp1 ==
  PS-Simulink Converter1 : nesl_utility/PS-Simulink Converter  PhysicalDomain=network_engine_domain  SubClassName=ps_output  LeftPortType=input  RightPortType=output  PseudoPeriodic=off  Frequencies=[]  VectorFormat=1-D array  Unit=deg  AffineConversion=off
  q : PMIOPort  Side=Left
  tag scope: q=global
  wires:
  PS-Simulink Converter1/1 -> [q]
  connections:
  PS-Simulink Converter1/LConn1 -- q/RConn1

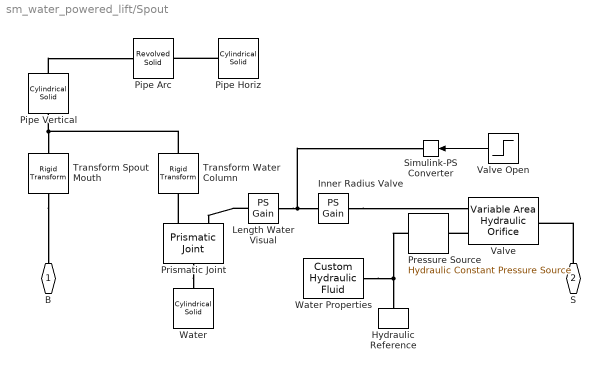
== system sm_water_powered_lift/Spout ==
  Hydraulic Reference : fl_lib/Hydraulic/Hydraulic Elements/Hydraulic Reference
  "Inner Radius Valve " : fl_lib/Physical Signals/Functions/PS Gain  gain=1.2*pi*(wrat.spout.water_col.radius)^2 m^2
  Length Water Visual : fl_lib/Physical Signals/Functions/PS Gain  gain=-wrat.spout.water_col.length m
  Pipe Vertical : sm_lib/Body Elements/Cylindrical Solid  CylinderRadius=wrat.spout.radius  CylinderRadiusUnits=m  CylinderLength=wrat.spout.pipe_length_1  CylinderLengthUnits=m  ExportEntireGeometry=off  InertiaType=CalculateFromGeometry  BasedOnType=Density  Density=1000  DensityUnits=kg/m^3  Mass=1  MassUnits=kg  CenterOfMass=[0 0 0]  CenterOfMassUnits=m  MomentsOfInertia=[1 1 1]  MomentsOfInertiaUnits=kg*m^2  ProductsOfInertia=[1 1 1]  ProductsOfInertiaUnits=kg*m^2  GraphicType=FromGeometry  MarkerShape=Sphere  MarkerSize=10  GraphicVisPropType=SimpleVisualProperties  GraphicDiffuseColor=[0.5 0.5 0.5]  GraphicOpacity=1  GraphicSpecularColor=[0.5 0.5 0.5 1.0]  GraphicAmbientColor=[0.15 0.15 0.15 1.0]  GraphicEmissiveColor=[0.0 0.0 0.0 1.0]  GraphicShininess=75  DoExposeReferenceFrame=off  SerializedFrames=<Frames><Frame><Id>Frame1</Id><Value><Name>F</Name><Origin><Source>GeometricFeature</Source><FeatureName>top surface</FeatureName></Origin><PrimaryAxis><DefinedDirection>+Z</DefinedDirection><Source>ReferenceFrame</Source><SourceDirection>+Z</SourceDirection><FeatureName></FeatureName></PrimaryAxis><SecondaryAxis><DefinedDirection>+X</DefinedDirection><Source>ReferenceFrame</Source><SourceDirection>+X</SourceDirection><FeatureName></FeatureName></SecondaryAxis></Value></Frame><Frame><Id>Frame2</Id><Value><Name>B</Name><Origin><Source>GeometricFeature</Source><FeatureName>bottom surface</FeatureName></Origin><PrimaryAxis><DefinedDirection>+Z</DefinedDirection><Source>ReferenceFrame</Source><SourceDirection>+Z</SourceDirection><FeatureName></FeatureName></PrimaryAxis><SecondaryAxis><DefinedDirection>+X</DefinedDirection><Source>ReferenceFrame</Source><SourceDirection>+X</SourceDirection><FeatureName></FeatureName></SecondaryAxis></Value></Frame></Frames>
  Pipe Arc : sm_lib/Body Elements/Revolved Solid  RevolutionCrossSection=wrat.spout.xc_data  RevolutionCrossSectionUnits=m  RevolutionExtent=Custom  RevolutionAngle=90  RevolutionAngleUnits=deg  ExportConvexHullGeometry=off  InertiaType=CalculateFromGeometry  BasedOnType=Density  Density=1000  DensityUnits=kg/m^3  Mass=1  MassUnits=kg  CenterOfMass=[0 0 0]  CenterOfMassUnits=m  MomentsOfInertia=[1 1 1]  MomentsOfInertiaUnits=kg*m^2  ProductsOfInertia=[1 1 1]  ProductsOfInertiaUnits=kg*m^2  GraphicType=FromGeometry  MarkerShape=Sphere  MarkerSize=10  GraphicVisPropType=SimpleVisualProperties  GraphicDiffuseColor=[0.5 0.5 0.5]  GraphicOpacity=1  GraphicSpecularColor=[0.5 0.5 0.5 1.0]  GraphicAmbientColor=[0.15 0.15 0.15 1.0]  GraphicEmissiveColor=[0.0 0.0 0.0 1.0]  GraphicShininess=75  DoExposeReferenceFrame=off  SerializedFrames=<Frames><Frame><Id>Frame1</Id><Value><Name>B</Name><Origin><Source>GeometricFeature</Source><FeatureName>back surface</FeatureName></Origin><PrimaryAxis><DefinedDirection>-Z</DefinedDirection><Source>GeometricFeature</Source><SourceDirection>+Z</SourceDirection><FeatureName>back surface</FeatureName></PrimaryAxis><SecondaryAxis><DefinedDirection>+X</DefinedDirection><Source>ReferenceFrame</Source><SourceDirection>+X</SourceDirection><FeatureName></FeatureName></SecondaryAxis></Value></Frame><Frame><Id>Frame2</Id><Value><Name>F</Name><Origin><Source>GeometricFeature</Source><FeatureName>front surface</FeatureName></Origin><PrimaryAxis><DefinedDirection>-Z</DefinedDirection><Source>GeometricFeature</Source><SourceDirection>+Z</SourceDirection><FeatureName>front surface</FeatureName></PrimaryAxis><SecondaryAxis><DefinedDirection>+X</DefinedDirection><Source>ReferenceFrame</Source><SourceDirection>+X</SourceDirection><FeatureName></FeatureName></SecondaryAxis></Value></Frame></Frames>
  Pipe Horiz : sm_lib/Body Elements/Cylindrical Solid  CylinderRadius=wrat.spout.radius  CylinderRadiusUnits=m  CylinderLength=wrat.spout.pipe_length_2  CylinderLengthUnits=m  ExportEntireGeometry=off  InertiaType=CalculateFromGeometry  BasedOnType=Density  Density=1000  DensityUnits=kg/m^3  Mass=1  MassUnits=kg  CenterOfMass=[0 0 0]  CenterOfMassUnits=m  MomentsOfInertia=[1 1 1]  MomentsOfInertiaUnits=kg*m^2  ProductsOfInertia=[1 1 1]  ProductsOfInertiaUnits=kg*m^2  GraphicType=FromGeometry  MarkerShape=Sphere  MarkerSize=10  GraphicVisPropType=SimpleVisualProperties  GraphicDiffuseColor=[0.5 0.5 0.5]  GraphicOpacity=1.0  GraphicSpecularColor=[0.5 0.5 0.5 1.0]  GraphicAmbientColor=[0.15 0.15 0.15 1.0]  GraphicEmissiveColor=[0.0 0.0 0.0 1.0]  GraphicShininess=75  DoExposeReferenceFrame=off  SerializedFrames=<Frames><Frame><Id>Frame1</Id><Value><Name>B</Name><Origin><Source>GeometricFeature</Source><FeatureName>top surface</FeatureName></Origin><PrimaryAxis><DefinedDirection>+Z</DefinedDirection><Source>ReferenceFrame</Source><SourceDirection>+Z</SourceDirection><FeatureName></FeatureName></PrimaryAxis><SecondaryAxis><DefinedDirection>+X</DefinedDirection><Source>ReferenceFrame</Source><SourceDirection>+X</SourceDirection><FeatureName></FeatureName></SecondaryAxis></Value></Frame></Frames>
  Pressure Source : fl_lib/Hydraulic/Hydraulic Sources/Hydraulic Constant Pressure Source  commanded_pressure=0.6*1000*9.81*8 Pa
  Prismatic Joint : sm_lib/Joints/Prismatic Joint  JointMode=Normal  CompositeWrenchDir=FollowerOnBase  CompositeWrenchFrame=BaseFrame  SenseConstraintForce=off  SenseConstraintTorque=off  SenseTotalForce=off  SenseTotalTorque=off  PositionTargetSpecify=off  PositionTargetPriority=High  PositionTargetValue=0  PositionTargetValueUnits=m  VelocityTargetSpecify=off  VelocityTargetPriority=High  VelocityTargetValue=0  VelocityTargetValueUnits=m/s  EquilibriumPosition=0  EquilibriumPositionUnits=m  SpringStiffness=0  SpringStiffnessUnits=N/m  DampingCoefficient=0  DampingCoefficientUnits=N/(m/s)  LowerLimitSpecify=off  LowerLimitBound=-1  LowerLimitBoundUnits=m  LowerLimitStiffness=1e6  LowerLimitStiffnessUnits=N/m  LowerLimitDamping=1e3  LowerLimitDampingUnits=N/(m/s)  LowerLimitTransitionRegionWidth=1e-4  LowerLimitTransitionRegionWidthUnits=m  UpperLimitSpecify=off  UpperLimitBound=1  UpperLimitBoundUnits=m  UpperLimitStiffness=1e6  UpperLimitStiffnessUnits=N/m  UpperLimitDamping=1e3  UpperLimitDampingUnits=N/(m/s)  UpperLimitTransitionRegionWidth=1e-4  UpperLimitTransitionRegionWidthUnits=m  TorqueActuationMode=ComputedTorque  MotionActuationMode=InputMotion  SensePosition=off  SenseVelocity=off  SenseAcceleration=off  SenseTorqueForce=off  SenseLowerLimitTorqueForce=off  SenseUpperLimitTorqueForce=off
  Simulink-PS Converter : nesl_utility/Simulink-PS Converter  PhysicalDomain=network_engine_domain  SubClassName=ps_input  LeftPortType=input  RightPortType=output  PseudoPeriodic=off  Frequencies=[]  NoiseDistribution=none  NoiseParameters=[]  Unit=1  AffineConversion=off  FilteringAndDerivatives=filter  SimscapeFilterOrder=2  InputFilterTimeConstant=0.1  UdotUserProvided=0
  Transform Spout Mouth : sm_lib/Frames and Transforms/Rigid Transform  RotationMethod=StandardAxis  FollAlignAxisA=+X  BaseAlignAxisA=+Y  FollAlignAxisB=+Y  BaseAlignAxisB=+Z  RotationStandardAxis=+Z  RotationAngle=180  RotationAngleUnits=deg  RotationArbitraryAxis=[0 0 1]  RotationSequenceAxes=FollowerAxes  RotationSequence=XYX  RotationSequenceAngles=[0 0 0]  RotationSequenceAnglesUnits=deg  RotationMatrix=[1 0 0; 0 1 0; 0 0 1]  Quaternion=[1 0 0 0]  TranslationMethod=Cartesian  TranslationCartesianOffset=[0 wrat.spout.offset_y*0.75 wrat.spout.offset_z*0.9]  TranslationCartesianOffsetUnits=m  TranslationStandardAxis=+Z  TranslationStandardOffset=0  TranslationStandardOffsetUnits=m  TranslationROffset=0  TranslationROffsetUnits=m  TranslationThetaOffset=0  TranslationThetaOffsetUnits=deg  TranslationZOffset=0  TranslationZOffsetUnits=m
  Transform Water Column : sm_lib/Frames and Transforms/Rigid Transform  RotationMethod=None  FollAlignAxisA=+X  BaseAlignAxisA=+Y  FollAlignAxisB=+Y  BaseAlignAxisB=+Z  RotationStandardAxis=+Z  RotationAngle=0.0  RotationAngleUnits=deg  RotationArbitraryAxis=[0 0 1]  RotationSequenceAxes=FollowerAxes  RotationSequence=XYX  RotationSequenceAngles=[0 0 0]  RotationSequenceAnglesUnits=deg  RotationMatrix=[1 0 0; 0 1 0; 0 0 1]  Quaternion=[1 0 0 0]  TranslationMethod=StandardAxis  TranslationCartesianOffset=[0 0 0]  TranslationCartesianOffsetUnits=m  TranslationStandardAxis=+Z  TranslationStandardOffset=wrat.spout.pipe_length_1*0.95  TranslationStandardOffsetUnits=m  TranslationROffset=0  TranslationROffsetUnits=m  TranslationThetaOffset=0  TranslationThetaOffsetUnits=deg  TranslationZOffset=0  TranslationZOffsetUnits=m
  Valve : fl_lib/Hydraulic/Hydraulic Elements/Variable Area Hydraulic Orifice  C_d=0.7  min_area=1e-5 m^2  lam_spec=1  B_lam=0.999  Re_cr=12  q_specify=off  q_priority=None  q=0.001 m^3/s  q_nominal_specify=off  q_nominal_value=1  q_nominal_unit=m^3/s  p_specify=off  p_priority=None  p=0 Pa  p_nominal_specify=off  p_nominal_value=1  p_nominal_unit=Pa
  Valve Open : Step  Time=0.1  SampleTime=0
  Water : sm_lib/Body Elements/Cylindrical Solid  CylinderRadius=wrat.spout.water_col.radius  CylinderRadiusUnits=m  CylinderLength=wrat.spout.water_col.length  CylinderLengthUnits=m  ExportEntireGeometry=off  InertiaType=CalculateFromGeometry  BasedOnType=Density  Density=1000  DensityUnits=kg/m^3  Mass=1  MassUnits=kg  CenterOfMass=[0 0 0]  CenterOfMassUnits=m  MomentsOfInertia=[1 1 1]  MomentsOfInertiaUnits=kg*m^2  ProductsOfInertia=[1 1 1]  ProductsOfInertiaUnits=kg*m^2  GraphicType=FromGeometry  MarkerShape=Sphere  MarkerSize=10  GraphicVisPropType=SimpleVisualProperties  GraphicDiffuseColor=wrat.water.clr  GraphicOpacity=wrat.water.opc  GraphicSpecularColor=[0.5 0.5 0.5 1.0]  GraphicAmbientColor=[0.15 0.15 0.15 1.0]  GraphicEmissiveColor=[0.0 0.0 0.0 1.0]  GraphicShininess=75  DoExposeReferenceFrame=on  SerializedFrames=<Frames/>
  Water Properties : fl_lib/Hydraulic/Hydraulic Utilities/Custom Hydraulic Fluid  density=1000 kg/m^3  viscosity_kin=1.004e-6 m^2/s  bulk=2.15e9 Pa  alpha=0.005  range_error=2  suppress_warning=false
  B : PMIOPort  Side=Left
  S : PMIOPort  Port=2  Side=Left
  wires:
  Valve Open/1 -> Simulink-PS Converter/1
  connections:
  Transform Spout Mouth/LConn1 -- B/RConn1
  Transform Water Column/LConn1 -- Transform Spout Mouth/RConn1 -- Pipe Vertical/RConn1
  Pipe Horiz/LConn1 -- Pipe Arc/RConn1
  Prismatic Joint/RConn1 -- Water/RConn1
  S/RConn1 -- Valve/RConn1
  Valve/LConn2 -- Pressure Source/LConn1
  Length Water Visual/RConn1 -- Prismatic Joint/LConn2
  Length Water Visual/LConn1 -- Simulink-PS Converter/RConn1 -- "Inner Radius Valve "/LConn1
  "Inner Radius Valve "/RConn1 -- Valve/LConn1
  Prismatic Joint/LConn1 -- Transform Water Column/RConn1
  Pressure Source/RConn1 -- Hydraulic Reference/LConn1 -- Water Properties/RConn1
  Pipe Vertical/LConn1 -- Pipe Arc/LConn1
